simulink model "Simulink_Control_BlueROV_Modo_Deslizante"  (R2019a)
settings: Solver=VariableStepAuto  StartTime=0.0  StopTime=100*3  RelTol=1e-3
values from neighbouring files (symbols this model uses):
  a0 = 50    [Control_BlueROV_Modo_Deslizante.m]
  a1 = 1    [Control_BlueROV_Modo_Deslizante.m]
  B = 78.38    [Control_BlueROV_Modo_Deslizante.m]
  eta = 1    [Control_BlueROV_Modo_Deslizante.m]
  Ix = 0.16    [Control_BlueROV_Modo_Deslizante.m]
  Ixy = 0    [Control_BlueROV_Modo_Deslizante.m]
  Ixz = 0    [Control_BlueROV_Modo_Deslizante.m]
  Iy = 0.16    [Control_BlueROV_Modo_Deslizante.m]
  Iyz = 0    [Control_BlueROV_Modo_Deslizante.m]
  Iz = 0.16    [Control_BlueROV_Modo_Deslizante.m]
  Kp = -0.07    [Control_BlueROV_Modo_Deslizante.m]
  Kpdot = -0.12    [Control_BlueROV_Modo_Deslizante.m]
  Kpp = -1.55    [Control_BlueROV_Modo_Deslizante.m]
  m = 7.31    [Control_BlueROV_Modo_Deslizante.m]
  M = Mrb+Ma    [Control_BlueROV_Modo_Deslizante.m]
  Minv = inv(M)    [Control_BlueROV_Modo_Deslizante.m]
  Mq = -0.07    [Control_BlueROV_Modo_Deslizante.m]
  Mqdot = -0.12    [Control_BlueROV_Modo_Deslizante.m]
  Mqq = -1.55    [Control_BlueROV_Modo_Deslizante.m]
  Nr = -0.07    [Control_BlueROV_Modo_Deslizante.m]
  Nrdot = -0.12    [Control_BlueROV_Modo_Deslizante.m]
  Nrr = -1.55    [Control_BlueROV_Modo_Deslizante.m]
  W = 71.71    [Control_BlueROV_Modo_Deslizante.m]
  xb = 0    [Control_BlueROV_Modo_Deslizante.m]
  xg = 0    [Control_BlueROV_Modo_Deslizante.m]
  Xu = -4.03    [Control_BlueROV_Modo_Deslizante.m]
  Xudot = -5.5    [Control_BlueROV_Modo_Deslizante.m]
  Xuu = -18.18    [Control_BlueROV_Modo_Deslizante.m]
  yb = 0    [Control_BlueROV_Modo_Deslizante.m]
  yg = 0    [Control_BlueROV_Modo_Deslizante.m]
  Yv = -6.22    [Control_BlueROV_Modo_Deslizante.m]
  Yvdot = -12.7    [Control_BlueROV_Modo_Deslizante.m]
  Yvv = -21.66    [Control_BlueROV_Modo_Deslizante.m]
  zb = 0.00019    [Control_BlueROV_Modo_Deslizante.m]
  zg = 0    [Control_BlueROV_Modo_Deslizante.m]
  Zw = -5.18    [Control_BlueROV_Modo_Deslizante.m]
  Zwdot = -14.57    [Control_BlueROV_Modo_Deslizante.m]
  Zww = -36.99    [Control_BlueROV_Modo_Deslizante.m]
(part 2 of 2)

== system Simulink_Control_BlueROV_Modo_Deslizante/BlueRov2/C(v)/Subsystem22 ==
  In1 : Inport
  In2 : Inport  Port=2
  In3 : Inport  Port=3
  In4 : Inport  Port=4
  Add4 : Sum  Inputs=+++
  Add8 : Sum
  Constant : Constant  Value=-Iyz
  Constant1 : Constant  Value=Iy
  Constant10 : Constant  Value=-Ixy
  Constant11 : Constant  Value=-Mqdot
  Product{1,19..21} (4 alike) : Product
  Out1 : Outport
  wires:
  In2/1 -> Product20/2
  In1/1 -> Product19/2
  Add8/1 -> Out1/1
  Constant10/1 -> Product20/1
  Product21/1 -> Add8/2
  Constant/1 -> Product19/1
  Product19/1 -> Add4/1
  Add4/1 -> Add8/1
  Constant11/1 -> Product21/1
  Product20/1 -> Add4/2
  Product1/1 -> Add4/3
  Constant1/1 -> Product1/1
  In4/1 -> Product21/2
  In3/1 -> Product1/2

== system Simulink_Control_BlueROV_Modo_Deslizante/BlueRov2/C(v)/Subsystem23 ==
  In1 : Inport
  In2 : Inport  Port=2
  In3 : Inport  Port=3
  In4 : Inport  Port=4
  Add4 : Sum  Inputs=+++
  Add8 : Sum
  Constant : Constant  Value=Ixz
  Constant1 : Constant  Value=-Ix
  Constant10 : Constant  Value=Ixy
  Constant11 : Constant  Value=Kpdot
  Product{1,19..21} (4 alike) : Product
  Out1 : Outport
  wires:
  In3/1 -> Product1/2
  In4/1 -> Product21/2
  Constant1/1 -> Product1/1
  Product1/1 -> Add4/3
  Product20/1 -> Add4/2
  Constant11/1 -> Product21/1
  Add4/1 -> Add8/1
  Product19/1 -> Add4/1
  Constant/1 -> Product19/1
  Product21/1 -> Add8/2
  Constant10/1 -> Product20/1
  Add8/1 -> Out1/1
  In1/1 -> Product19/2
  In2/1 -> Product20/2

== system Simulink_Control_BlueROV_Modo_Deslizante/BlueRov2/C(v)/Subsystem3 ==
  In1 : Inport
  In2 : Inport  Port=2
  In3 : Inport  Port=3
  Add4 : Sum
  Add8 : Sum  Inputs=-+
  Constant : Constant  Value=yg
  Constant10 : Constant
  Constant11 : Constant  Value=Zwdot
  Gain : Gain  Gain=m
  Product19 : Product
  Product20 : Product
  Product21 : Product
  Out1 : Outport
  wires:
  In2/1 -> Product20/2
  In3/1 -> Product21/2
  In1/1 -> Product19/2
  Add8/1 -> Out1/1
  Constant10/1 -> Product20/1
  Add4/1 -> Gain/1
  Product21/1 -> Add8/2
  Constant/1 -> Product19/1
  Product19/1 -> Add4/1
  Gain/1 -> Add8/1
  Constant11/1 -> Product21/1
  Product20/1 -> Add4/2

== system Simulink_Control_BlueROV_Modo_Deslizante/BlueRov2/C(v)/Subsystem4 ==
  In1 : Inport
  In2 : Inport  Port=2
  Add4 : Sum
  Constant : Constant  Value=zg
  Constant10 : Constant  Value=xg
  Gain : Gain  Gain=m
  Product19 : Product
  Product20 : Product
  Out1 : Outport
  wires:
  In2/1 -> Product20/2
  Add4/1 -> Gain/1
  Constant10/1 -> Product20/1
  Gain/1 -> Out1/1
  Constant/1 -> Product19/1
  In1/1 -> Product19/2
  Product19/1 -> Add4/1
  Product20/1 -> Add4/2

== system Simulink_Control_BlueROV_Modo_Deslizante/BlueRov2/C(v)/Subsystem5 ==
  In1 : Inport
  In2 : Inport  Port=2
  In3 : Inport  Port=3
  Add4 : Sum  Inputs=+-
  Add8 : Sum  Inputs=-+
  Constant : Constant  Value=yg
  Constant10 : Constant
  Constant11 : Constant  Value=-Xudot
  Gain : Gain  Gain=m
  Product19 : Product
  Product20 : Product
  Product21 : Product
  Out1 : Outport
  wires:
  Product20/1 -> Add4/2
  Constant11/1 -> Product21/1
  Gain/1 -> Add8/1
  Product19/1 -> Add4/1
  Constant/1 -> Product19/1
  Product21/1 -> Add8/2
  Add4/1 -> Gain/1
  Constant10/1 -> Product20/1
  Add8/1 -> Out1/1
  In1/1 -> Product19/2
  In3/1 -> Product21/2
  In2/1 -> Product20/2

== system Simulink_Control_BlueROV_Modo_Deslizante/BlueRov2/C(v)/Subsystem6 ==
  In1 : Inport
  In2 : Inport  Port=2
  In3 : Inport  Port=3
  Add4 : Sum  Inputs=+-
  Add8 : Sum  Inputs=-+
  Constant : Constant  Value=zg
  Constant10 : Constant
  Constant11 : Constant  Value=-Yvdot
  Gain : Gain  Gain=m
  Product19 : Product
  Product20 : Product
  Product21 : Product
  Out1 : Outport
  wires:
  In2/1 -> Product20/2
  In3/1 -> Product21/2
  In1/1 -> Product19/2
  Add8/1 -> Out1/1
  Constant10/1 -> Product20/1
  Add4/1 -> Gain/1
  Product21/1 -> Add8/2
  Constant/1 -> Product19/1
  Product19/1 -> Add4/1
  Gain/1 -> Add8/1
  Constant11/1 -> Product21/1
  Product20/1 -> Add4/2

== system Simulink_Control_BlueROV_Modo_Deslizante/BlueRov2/C(v)/Subsystem7 ==
  In1 : Inport
  In2 : Inport  Port=2
  In3 : Inport  Port=3
  Add4 : Sum
  Add8 : Sum  Inputs=-+
  Constant : Constant  Value=zg
  Constant10 : Constant
  Constant11 : Constant  Value=Xudot
  Gain : Gain  Gain=m
  Product19 : Product
  Product20 : Product
  Product21 : Product
  Out1 : Outport
  wires:
  Product20/1 -> Add4/2
  Constant11/1 -> Product21/1
  Gain/1 -> Add8/1
  Product19/1 -> Add4/1
  Constant/1 -> Product19/1
  Product21/1 -> Add8/2
  Add4/1 -> Gain/1
  Constant10/1 -> Product20/1
  Add8/1 -> Out1/1
  In1/1 -> Product19/2
  In3/1 -> Product21/2
  In2/1 -> Product20/2

== system Simulink_Control_BlueROV_Modo_Deslizante/BlueRov2/C(v)/Subsystem8 ==
  In1 : Inport
  In2 : Inport  Port=2
  Add4 : Sum
  Constant : Constant  Value=xg
  Constant10 : Constant  Value=yg
  Gain : Gain  Gain=m
  Product19 : Product
  Product20 : Product
  Out1 : Outport
  wires:
  In2/1 -> Product20/2
  Add4/1 -> Gain/1
  Constant10/1 -> Product20/1
  Gain/1 -> Out1/1
  Constant/1 -> Product19/1
  In1/1 -> Product19/2
  Product19/1 -> Add4/1
  Product20/1 -> Add4/2

== system Simulink_Control_BlueROV_Modo_Deslizante/BlueRov2/C(v)/Subsystem9 ==
  In1 : Inport
  In2 : Inport  Port=2
  Add4 : Sum
  Constant : Constant  Value=yg
  Constant10 : Constant  Value=zg
  Gain : Gain  Gain=-m
  Product19 : Product
  Product20 : Product
  Out1 : Outport
  wires:
  In2/1 -> Product20/2
  Add4/1 -> Gain/1
  Constant10/1 -> Product20/1
  Gain/1 -> Out1/1
  Constant/1 -> Product19/1
  In1/1 -> Product19/2
  Product19/1 -> Add4/1
  Product20/1 -> Add4/2

== system Simulink_Control_BlueROV_Modo_Deslizante/BlueRov2/J(n)/Subsystem1 ==
  In1 : Inport
  In2 : Inport  Port=2
  Product6 : Product
  Out1 : Outport
  wires:
  In1/1 -> Product6/1
  In2/1 -> Product6/2
  Product6/1 -> Out1/1

== system Simulink_Control_BlueROV_Modo_Deslizante/BlueRov2/J(n)/Subsystem10 ==
  In1 : Inport
  In2 : Inport  Port=2
  Product6 : Product
  Out1 : Outport
  wires:
  In1/1 -> Product6/1
  In2/1 -> Product6/2
  Product6/1 -> Out1/1

== system Simulink_Control_BlueROV_Modo_Deslizante/BlueRov2/J(n)/Subsystem11 ==
  In1 : Inport
  In2 : Inport  Port=2
  Product6 : Product
  Out1 : Outport
  wires:
  In1/1 -> Product6/1
  In2/1 -> Product6/2
  Product6/1 -> Out1/1

== system Simulink_Control_BlueROV_Modo_Deslizante/BlueRov2/J(n)/Subsystem12 ==
  In1 : Inport
  In2 : Inport  Port=2
  Product6 : Product
  Out1 : Outport
  wires:
  In1/1 -> Product6/1
  In2/1 -> Product6/2
  Product6/1 -> Out1/1

== system Simulink_Control_BlueROV_Modo_Deslizante/BlueRov2/J(n)/Subsystem2 ==
  In1 : Inport
  In2 : Inport  Port=2
  In3 : Inport  Port=3
  In4 : Inport  Port=4
  In5 : Inport  Port=5
  Add7 : Sum
  Product37 : Product
  Product38 : Product  Inputs=3
  Out1 : Outport
  wires:
  In5/1 -> Product38/3
  In4/1 -> Product38/2
  In3/1 -> Product38/1
  In2/1 -> Product37/2
  In1/1 -> Product37/1
  Product37/1 -> Add7/1
  Add7/1 -> Out1/1
  Product38/1 -> Add7/2

== system Simulink_Control_BlueROV_Modo_Deslizante/BlueRov2/J(n)/Subsystem3 ==
  In1 : Inport
  In2 : Inport  Port=2
  Product6 : Product
  Out1 : Outport
  wires:
  Product6/1 -> Out1/1
  In2/1 -> Product6/2
  In1/1 -> Product6/1

== system Simulink_Control_BlueROV_Modo_Deslizante/BlueRov2/J(n)/Subsystem4 ==
  In1 : Inport
  In2 : Inport  Port=2
  In3 : Inport  Port=3
  In4 : Inport  Port=4
  In5 : Inport  Port=5
  Add7 : Sum  Inputs=-+
  Product37 : Product
  Product38 : Product  Inputs=3
  Out1 : Outport
  wires:
  Product38/1 -> Add7/2
  Add7/1 -> Out1/1
  Product37/1 -> Add7/1
  In1/1 -> Product37/1
  In2/1 -> Product37/2
  In3/1 -> Product38/1
  In4/1 -> Product38/2
  In5/1 -> Product38/3

== system Simulink_Control_BlueROV_Modo_Deslizante/BlueRov2/J(n)/Subsystem5 ==
  In1 : Inport
  In2 : Inport  Port=2
  In3 : Inport  Port=3
  In4 : Inport  Port=4
  In5 : Inport  Port=5
  Add7 : Sum
  Product37 : Product
  Product38 : Product  Inputs=3
  Out1 : Outport
  wires:
  Product38/1 -> Add7/2
  Add7/1 -> Out1/1
  Product37/1 -> Add7/1
  In1/1 -> Product37/1
  In2/1 -> Product37/2
  In3/1 -> Product38/1
  In4/1 -> Product38/2
  In5/1 -> Product38/3

== system Simulink_Control_BlueROV_Modo_Deslizante/BlueRov2/J(n)/Subsystem6 ==
  In1 : Inport
  In2 : Inport  Port=2
  In3 : Inport  Port=3
  In4 : Inport  Port=4
  In5 : Inport  Port=5
  Add7 : Sum  Inputs=-+
  Product37 : Product
  Product38 : Product  Inputs=3
  Out1 : Outport
  wires:
  In5/1 -> Product38/3
  In4/1 -> Product38/2
  In3/1 -> Product38/1
  In2/1 -> Product37/2
  In1/1 -> Product37/1
  Product37/1 -> Add7/1
  Add7/1 -> Out1/1
  Product38/1 -> Add7/2

== system Simulink_Control_BlueROV_Modo_Deslizante/BlueRov2/J(n)/Subsystem7 ==
  In1 : Inport
  In2 : Inport  Port=2
  Product6 : Product
  Out1 : Outport
  wires:
  In1/1 -> Product6/1
  In2/1 -> Product6/2
  Product6/1 -> Out1/1

== system Simulink_Control_BlueROV_Modo_Deslizante/BlueRov2/J(n)/Subsystem8 ==
  In1 : Inport
  In2 : Inport  Port=2
  Product6 : Product
  Out1 : Outport
  wires:
  Product6/1 -> Out1/1
  In2/1 -> Product6/2
  In1/1 -> Product6/1

== system Simulink_Control_BlueROV_Modo_Deslizante/BlueRov2/J(n)/Subsystem9 ==
  In1 : Inport
  In2 : Inport  Port=2
  Product6 : Product
  Out1 : Outport
  wires:
  In1/1 -> Product6/1
  In2/1 -> Product6/2
  Product6/1 -> Out1/1

== system Simulink_Control_BlueROV_Modo_Deslizante/Estimador de Variable/C(v)/Subsystem ==
  In1 : Inport
  In2 : Inport  Port=2
  Add4 : Sum
  Constant : Constant  Value=zg
  Constant10 : Constant  Value=yg
  Gain : Gain  Gain=m
  Product19 : Product
  Product20 : Product
  Out1 : Outport
  wires:
  Product20/1 -> Add4/2
  Product19/1 -> Add4/1
  In1/1 -> Product19/2
  Constant/1 -> Product19/1
  Gain/1 -> Out1/1
  Constant10/1 -> Product20/1
  Add4/1 -> Gain/1
  In2/1 -> Product20/2

== system Simulink_Control_BlueROV_Modo_Deslizante/Estimador de Variable/C(v)/Subsystem1 ==
  In1 : Inport
  In2 : Inport  Port=2
  In3 : Inport  Port=3
  Add4 : Sum  Inputs=+-
  Add8 : Sum  Inputs=-+
  Constant : Constant  Value=xg
  Constant10 : Constant
  Constant11 : Constant  Value=-Zwdot
  Gain : Gain  Gain=m
  Product19 : Product
  Product20 : Product
  Product21 : Product
  Out1 : Outport
  wires:
  Product20/1 -> Add4/2
  Constant11/1 -> Product21/1
  Gain/1 -> Add8/1
  Product19/1 -> Add4/1
  Constant/1 -> Product19/1
  Product21/1 -> Add8/2
  Add4/1 -> Gain/1
  Constant10/1 -> Product20/1
  Add8/1 -> Out1/1
  In1/1 -> Product19/2
  In3/1 -> Product21/2
  In2/1 -> Product20/2

== system Simulink_Control_BlueROV_Modo_Deslizante/Estimador de Variable/C(v)/Subsystem10 ==
  In1 : Inport
  In2 : Inport  Port=2
  In3 : Inport  Port=3
  Add4 : Sum
  Add8 : Sum
  Constant : Constant  Value=yg
  Constant10 : Constant
  Constant11 : Constant  Value=-Zwdot
  Gain : Gain  Gain=m
  Product19 : Product
  Product20 : Product
  Product21 : Product
  Out1 : Outport
  wires:
  In2/1 -> Product20/2
  In3/1 -> Product21/2
  In1/1 -> Product19/2
  Add8/1 -> Out1/1
  Constant10/1 -> Product20/1
  Add4/1 -> Gain/1
  Product21/1 -> Add8/2
  Constant/1 -> Product19/1
  Product19/1 -> Add4/1
  Gain/1 -> Add8/1
  Constant11/1 -> Product21/1
  Product20/1 -> Add4/2

== system Simulink_Control_BlueROV_Modo_Deslizante/Estimador de Variable/C(v)/Subsystem11 ==
  In1 : Inport
  In2 : Inport  Port=2
  In3 : Inport  Port=3
  Add4 : Sum  Inputs=+-
  Add8 : Sum
  Constant : Constant  Value=zg
  Constant10 : Constant
  Constant11 : Constant  Value=Yvdot
  Gain : Gain  Gain=m
  Product19 : Product
  Product20 : Product
  Product21 : Product
  Out1 : Outport
  wires:
  Product20/1 -> Add4/2
  Constant11/1 -> Product21/1
  Gain/1 -> Add8/1
  Product19/1 -> Add4/1
  Constant/1 -> Product19/1
  Product21/1 -> Add8/2
  Add4/1 -> Gain/1
  Constant10/1 -> Product20/1
  Add8/1 -> Out1/1
  In1/1 -> Product19/2
  In3/1 -> Product21/2
  In2/1 -> Product20/2

== system Simulink_Control_BlueROV_Modo_Deslizante/Estimador de Variable/C(v)/Subsystem12 ==
  In1 : Inport
  In2 : Inport  Port=2
  In3 : Inport  Port=3
  In4 : Inport  Port=4
  Add4 : Sum  Inputs=+++
  Add8 : Sum
  Constant : Constant  Value=-Iyz
  Constant1 : Constant  Value=Iz
  Constant10 : Constant  Value=-Ixz
  Constant11 : Constant  Value=-Nrdot
  Product{1,19..21} (4 alike) : Product
  Out1 : Outport
  wires:
  In2/1 -> Product20/2
  In1/1 -> Product19/2
  Add8/1 -> Out1/1
  Constant10/1 -> Product20/1
  Product21/1 -> Add8/2
  Constant/1 -> Product19/1
  Product19/1 -> Add4/1
  Add4/1 -> Add8/1
  Constant11/1 -> Product21/1
  Product20/1 -> Add4/2
  Product1/1 -> Add4/3
  Constant1/1 -> Product1/1
  In4/1 -> Product21/2
  In3/1 -> Product1/2

== system Simulink_Control_BlueROV_Modo_Deslizante/Estimador de Variable/C(v)/Subsystem13 ==
  In1 : Inport
  In2 : Inport  Port=2
  In3 : Inport  Port=3
  In4 : Inport  Port=4
  Add4 : Sum  Inputs=+++
  Add8 : Sum
  Constant : Constant  Value=Iyz
  Constant1 : Constant  Value=-Iy
  Constant10 : Constant  Value=Ixy
  Constant11 : Constant  Value=Mqdot
  Product{1,19..21} (4 alike) : Product
  Out1 : Outport
  wires:
  In3/1 -> Product1/2
  In4/1 -> Product21/2
  Constant1/1 -> Product1/1
  Product1/1 -> Add4/3
  Product20/1 -> Add4/2
  Constant11/1 -> Product21/1
  Add4/1 -> Add8/1
  Product19/1 -> Add4/1
  Constant/1 -> Product19/1
  Product21/1 -> Add8/2
  Constant10/1 -> Product20/1
  Add8/1 -> Out1/1
  In1/1 -> Product19/2
  In2/1 -> Product20/2

== system Simulink_Control_BlueROV_Modo_Deslizante/Estimador de Variable/C(v)/Subsystem14 ==
  In1 : Inport
  In2 : Inport  Port=2
  In3 : Inport  Port=3
  Add4 : Sum  Inputs=+-
  Add8 : Sum
  Constant : Constant  Value=xg
  Constant10 : Constant
  Constant11 : Constant  Value=Zwdot
  Gain : Gain  Gain=m
  Product19 : Product
  Product20 : Product
  Product21 : Product
  Out1 : Outport
  wires:
  Product20/1 -> Add4/2
  Constant11/1 -> Product21/1
  Gain/1 -> Add8/1
  Product19/1 -> Add4/1
  Constant/1 -> Product19/1
  Product21/1 -> Add8/2
  Add4/1 -> Gain/1
  Constant10/1 -> Product20/1
  Add8/1 -> Out1/1
  In1/1 -> Product19/2
  In3/1 -> Product21/2
  In2/1 -> Product20/2

== system Simulink_Control_BlueROV_Modo_Deslizante/Estimador de Variable/C(v)/Subsystem15 ==
  In1 : Inport
  In2 : Inport  Port=2
  In3 : Inport  Port=3
  Add4 : Sum
  Add8 : Sum
  Constant : Constant  Value=zg
  Constant10 : Constant
  Constant11 : Constant  Value=-Xudot
  Gain : Gain  Gain=m
  Product19 : Product
  Product20 : Product
  Product21 : Product
  Out1 : Outport
  wires:
  In2/1 -> Product20/2
  In3/1 -> Product21/2
  In1/1 -> Product19/2
  Add8/1 -> Out1/1
  Constant10/1 -> Product20/1
  Add4/1 -> Gain/1
  Product21/1 -> Add8/2
  Constant/1 -> Product19/1
  Product19/1 -> Add4/1
  Gain/1 -> Add8/1
  Constant11/1 -> Product21/1
  Product20/1 -> Add4/2

== system Simulink_Control_BlueROV_Modo_Deslizante/Estimador de Variable/C(v)/Subsystem16 ==
  In1 : Inport
  In2 : Inport  Port=2
  Add4 : Sum
  Constant : Constant  Value=zg
  Constant10 : Constant  Value=xg
  Gain : Gain  Gain=-m
  Product19 : Product
  Product20 : Product
  Out1 : Outport
  wires:
  Product20/1 -> Add4/2
  Product19/1 -> Add4/1
  In1/1 -> Product19/2
  Constant/1 -> Product19/1
  Gain/1 -> Out1/1
  Constant10/1 -> Product20/1
  Add4/1 -> Gain/1
  In2/1 -> Product20/2

== system Simulink_Control_BlueROV_Modo_Deslizante/Estimador de Variable/C(v)/Subsystem17 ==
  In1 : Inport
  In2 : Inport  Port=2
  In3 : Inport  Port=3
  In4 : Inport  Port=4
  Add4 : Sum  Inputs=+++
  Add8 : Sum
  Constant : Constant  Value=Iyz
  Constant1 : Constant  Value=-Iz
  Constant10 : Constant  Value=Ixz
  Constant11 : Constant  Value=Nrdot
  Product{1,19..21} (4 alike) : Product
  Out1 : Outport
  wires:
  In3/1 -> Product1/2
  In4/1 -> Product21/2
  Constant1/1 -> Product1/1
  Product1/1 -> Add4/3
  Product20/1 -> Add4/2
  Constant11/1 -> Product21/1
  Add4/1 -> Add8/1
  Product19/1 -> Add4/1
  Constant/1 -> Product19/1
  Product21/1 -> Add8/2
  Constant10/1 -> Product20/1
  Add8/1 -> Out1/1
  In1/1 -> Product19/2
  In2/1 -> Product20/2

== system Simulink_Control_BlueROV_Modo_Deslizante/Estimador de Variable/C(v)/Subsystem18 ==
  In1 : Inport
  In2 : Inport  Port=2
  In3 : Inport  Port=3
  In4 : Inport  Port=4
  Add4 : Sum  Inputs=+++
  Add8 : Sum
  Constant : Constant  Value=-Ixz
  Constant1 : Constant  Value=Ix
  Constant10 : Constant  Value=-Ixy
  Constant11 : Constant  Value=-Kpdot
  Product{1,19..21} (4 alike) : Product
  Out1 : Outport
  wires:
  In2/1 -> Product20/2
  In1/1 -> Product19/2
  Add8/1 -> Out1/1
  Constant10/1 -> Product20/1
  Product21/1 -> Add8/2
  Constant/1 -> Product19/1
  Product19/1 -> Add4/1
  Add4/1 -> Add8/1
  Constant11/1 -> Product21/1
  Product20/1 -> Add4/2
  Product1/1 -> Add4/3
  Constant1/1 -> Product1/1
  In4/1 -> Product21/2
  In3/1 -> Product1/2

== system Simulink_Control_BlueROV_Modo_Deslizante/Estimador de Variable/C(v)/Subsystem19 ==
  In1 : Inport
  In2 : Inport  Port=2
  In3 : Inport  Port=3
  Add4 : Sum
  Add8 : Sum
  Constant : Constant  Value=xg
  Constant10 : Constant
  Constant11 : Constant  Value=-Yvdot
  Gain : Gain  Gain=m
  Product19 : Product
  Product20 : Product
  Product21 : Product
  Out1 : Outport
  wires:
  In2/1 -> Product20/2
  In3/1 -> Product21/2
  In1/1 -> Product19/2
  Add8/1 -> Out1/1
  Constant10/1 -> Product20/1
  Add4/1 -> Gain/1
  Product21/1 -> Add8/2
  Constant/1 -> Product19/1
  Product19/1 -> Add4/1
  Gain/1 -> Add8/1
  Constant11/1 -> Product21/1
  Product20/1 -> Add4/2

== system Simulink_Control_BlueROV_Modo_Deslizante/Estimador de Variable/C(v)/Subsystem2 ==
  In1 : Inport
  In2 : Inport  Port=2
  In3 : Inport  Port=3
  Add10 : Sum  Inputs=-+
  Add9 : Sum
  Constant12 : Constant  Value=xg
  Constant13 : Constant
  Constant14 : Constant  Value=Yvdot
  Gain1 : Gain  Gain=m
  Product22 : Product
  Product23 : Product
  Product24 : Product
  Out1 : Outport
  wires:
  In1/1 -> Product22/2
  Constant14/1 -> Product24/1
  Add9/1 -> Gain1/1
  Constant12/1 -> Product22/1
  Product23/1 -> Add9/2
  Gain1/1 -> Add10/1
  Constant13/1 -> Product23/1
  Product24/1 -> Add10/2
  Product22/1 -> Add9/1
  In3/1 -> Product24/2
  Add10/1 -> Out1/1
  In2/1 -> Product23/2

== system Simulink_Control_BlueROV_Modo_Deslizante/Estimador de Variable/C(v)/Subsystem20 ==
  In1 : Inport
  In2 : Inport  Port=2
  In3 : Inport  Port=3
  Add4 : Sum
  Add8 : Sum
  Constant : Constant  Value=yg
  Constant10 : Constant  Value=-1
  Constant11 : Constant  Value=Xudot
  Gain : Gain  Gain=m
  Product19 : Product
  Product20 : Product
  Product21 : Product
  Out1 : Outport
  wires:
  Product20/1 -> Add4/2
  Constant11/1 -> Product21/1
  Gain/1 -> Add8/1
  Product19/1 -> Add4/1
  Constant/1 -> Product19/1
  Product21/1 -> Add8/2
  Add4/1 -> Gain/1
  Constant10/1 -> Product20/1
  Add8/1 -> Out1/1
  In1/1 -> Product19/2
  In3/1 -> Product21/2
  In2/1 -> Product20/2

== system Simulink_Control_BlueROV_Modo_Deslizante/Estimador de Variable/C(v)/Subsystem21 ==
  In1 : Inport
  In2 : Inport  Port=2
  Add4 : Sum
  Constant : Constant  Value=xg
  Constant10 : Constant  Value=yg
  Gain : Gain  Gain=-m
  Product19 : Product
  Product20 : Product
  Out1 : Outport
  wires:
  In2/1 -> Product20/2
  Add4/1 -> Gain/1
  Constant10/1 -> Product20/1
  Gain/1 -> Out1/1
  Constant/1 -> Product19/1
  In1/1 -> Product19/2
  Product19/1 -> Add4/1
  Product20/1 -> Add4/2

== system Simulink_Control_BlueROV_Modo_Deslizante/Estimador de Variable/C(v)/Subsystem22 ==
  In1 : Inport
  In2 : Inport  Port=2
  In3 : Inport  Port=3
  In4 : Inport  Port=4
  Add4 : Sum  Inputs=+++
  Add8 : Sum
  Constant : Constant  Value=-Iyz
  Constant1 : Constant  Value=Iy
  Constant10 : Constant  Value=-Ixy
  Constant11 : Constant  Value=-Mqdot
  Product{1,19..21} (4 alike) : Product
  Out1 : Outport
  wires:
  In2/1 -> Product20/2
  In1/1 -> Product19/2
  Add8/1 -> Out1/1
  Constant10/1 -> Product20/1
  Product21/1 -> Add8/2
  Constant/1 -> Product19/1
  Product19/1 -> Add4/1
  Add4/1 -> Add8/1
  Constant11/1 -> Product21/1
  Product20/1 -> Add4/2
  Product1/1 -> Add4/3
  Constant1/1 -> Product1/1
  In4/1 -> Product21/2
  In3/1 -> Product1/2

== system Simulink_Control_BlueROV_Modo_Deslizante/Estimador de Variable/C(v)/Subsystem23 ==
  In1 : Inport
  In2 : Inport  Port=2
  In3 : Inport  Port=3
  In4 : Inport  Port=4
  Add4 : Sum  Inputs=+++
  Add8 : Sum
  Constant : Constant  Value=Ixz
  Constant1 : Constant  Value=-Ix
  Constant10 : Constant  Value=Ixy
  Constant11 : Constant  Value=Kpdot
  Product{1,19..21} (4 alike) : Product
  Out1 : Outport
  wires:
  In3/1 -> Product1/2
  In4/1 -> Product21/2
  Constant1/1 -> Product1/1
  Product1/1 -> Add4/3
  Product20/1 -> Add4/2
  Constant11/1 -> Product21/1
  Add4/1 -> Add8/1
  Product19/1 -> Add4/1
  Constant/1 -> Product19/1
  Product21/1 -> Add8/2
  Constant10/1 -> Product20/1
  Add8/1 -> Out1/1
  In1/1 -> Product19/2
  In2/1 -> Product20/2

== system Simulink_Control_BlueROV_Modo_Deslizante/Estimador de Variable/C(v)/Subsystem3 ==
  In1 : Inport
  In2 : Inport  Port=2
  In3 : Inport  Port=3
  Add4 : Sum
  Add8 : Sum  Inputs=-+
  Constant : Constant  Value=yg
  Constant10 : Constant
  Constant11 : Constant  Value=Zwdot
  Gain : Gain  Gain=m
  Product19 : Product
  Product20 : Product
  Product21 : Product
  Out1 : Outport
  wires:
  In2/1 -> Product20/2
  In3/1 -> Product21/2
  In1/1 -> Product19/2
  Add8/1 -> Out1/1
  Constant10/1 -> Product20/1
  Add4/1 -> Gain/1
  Product21/1 -> Add8/2
  Constant/1 -> Product19/1
  Product19/1 -> Add4/1
  Gain/1 -> Add8/1
  Constant11/1 -> Product21/1
  Product20/1 -> Add4/2

== system Simulink_Control_BlueROV_Modo_Deslizante/Estimador de Variable/C(v)/Subsystem4 ==
  In1 : Inport
  In2 : Inport  Port=2
  Add4 : Sum
  Constant : Constant  Value=zg
  Constant10 : Constant  Value=xg
  Gain : Gain  Gain=m
  Product19 : Product
  Product20 : Product
  Out1 : Outport
  wires:
  In2/1 -> Product20/2
  Add4/1 -> Gain/1
  Constant10/1 -> Product20/1
  Gain/1 -> Out1/1
  Constant/1 -> Product19/1
  In1/1 -> Product19/2
  Product19/1 -> Add4/1
  Product20/1 -> Add4/2

== system Simulink_Control_BlueROV_Modo_Deslizante/Estimador de Variable/C(v)/Subsystem5 ==
  In1 : Inport
  In2 : Inport  Port=2
  In3 : Inport  Port=3
  Add4 : Sum  Inputs=+-
  Add8 : Sum  Inputs=-+
  Constant : Constant  Value=yg
  Constant10 : Constant
  Constant11 : Constant  Value=-Xudot
  Gain : Gain  Gain=m
  Product19 : Product
  Product20 : Product
  Product21 : Product
  Out1 : Outport
  wires:
  Product20/1 -> Add4/2
  Constant11/1 -> Product21/1
  Gain/1 -> Add8/1
  Product19/1 -> Add4/1
  Constant/1 -> Product19/1
  Product21/1 -> Add8/2
  Add4/1 -> Gain/1
  Constant10/1 -> Product20/1
  Add8/1 -> Out1/1
  In1/1 -> Product19/2
  In3/1 -> Product21/2
  In2/1 -> Product20/2

== system Simulink_Control_BlueROV_Modo_Deslizante/Estimador de Variable/C(v)/Subsystem6 ==
  In1 : Inport
  In2 : Inport  Port=2
  In3 : Inport  Port=3
  Add4 : Sum  Inputs=+-
  Add8 : Sum  Inputs=-+
  Constant : Constant  Value=zg
  Constant10 : Constant
  Constant11 : Constant  Value=-Yvdot
  Gain : Gain  Gain=m
  Product19 : Product
  Product20 : Product
  Product21 : Product
  Out1 : Outport
  wires:
  In2/1 -> Product20/2
  In3/1 -> Product21/2
  In1/1 -> Product19/2
  Add8/1 -> Out1/1
  Constant10/1 -> Product20/1
  Add4/1 -> Gain/1
  Product21/1 -> Add8/2
  Constant/1 -> Product19/1
  Product19/1 -> Add4/1
  Gain/1 -> Add8/1
  Constant11/1 -> Product21/1
  Product20/1 -> Add4/2

== system Simulink_Control_BlueROV_Modo_Deslizante/Estimador de Variable/C(v)/Subsystem7 ==
  In1 : Inport
  In2 : Inport  Port=2
  In3 : Inport  Port=3
  Add4 : Sum
  Add8 : Sum  Inputs=-+
  Constant : Constant  Value=zg
  Constant10 : Constant
  Constant11 : Constant  Value=Xudot
  Gain : Gain  Gain=m
  Product19 : Product
  Product20 : Product
  Product21 : Product
  Out1 : Outport
  wires:
  Product20/1 -> Add4/2
  Constant11/1 -> Product21/1
  Gain/1 -> Add8/1
  Product19/1 -> Add4/1
  Constant/1 -> Product19/1
  Product21/1 -> Add8/2
  Add4/1 -> Gain/1
  Constant10/1 -> Product20/1
  Add8/1 -> Out1/1
  In1/1 -> Product19/2
  In3/1 -> Product21/2
  In2/1 -> Product20/2

== system Simulink_Control_BlueROV_Modo_Deslizante/Estimador de Variable/C(v)/Subsystem8 ==
  In1 : Inport
  In2 : Inport  Port=2
  Add4 : Sum
  Constant : Constant  Value=xg
  Constant10 : Constant  Value=yg
  Gain : Gain  Gain=m
  Product19 : Product
  Product20 : Product
  Out1 : Outport
  wires:
  In2/1 -> Product20/2
  Add4/1 -> Gain/1
  Constant10/1 -> Product20/1
  Gain/1 -> Out1/1
  Constant/1 -> Product19/1
  In1/1 -> Product19/2
  Product19/1 -> Add4/1
  Product20/1 -> Add4/2

== system Simulink_Control_BlueROV_Modo_Deslizante/Estimador de Variable/C(v)/Subsystem9 ==
  In1 : Inport
  In2 : Inport  Port=2
  Add4 : Sum
  Constant : Constant  Value=yg
  Constant10 : Constant  Value=zg
  Gain : Gain  Gain=-m
  Product19 : Product
  Product20 : Product
  Out1 : Outport
  wires:
  In2/1 -> Product20/2
  Add4/1 -> Gain/1
  Constant10/1 -> Product20/1
  Gain/1 -> Out1/1
  Constant/1 -> Product19/1
  In1/1 -> Product19/2
  Product19/1 -> Add4/1
  Product20/1 -> Add4/2

== system Simulink_Control_BlueROV_Modo_Deslizante/Estimador de Variable/J(n)/Subsystem1 ==
  In1 : Inport
  In2 : Inport  Port=2
  Product6 : Product
  Out1 : Outport
  wires:
  In1/1 -> Product6/1
  In2/1 -> Product6/2
  Product6/1 -> Out1/1

== system Simulink_Control_BlueROV_Modo_Deslizante/Estimador de Variable/J(n)/Subsystem10 ==
  In1 : Inport
  In2 : Inport  Port=2
  Product6 : Product
  Out1 : Outport
  wires:
  In1/1 -> Product6/1
  In2/1 -> Product6/2
  Product6/1 -> Out1/1

== system Simulink_Control_BlueROV_Modo_Deslizante/Estimador de Variable/J(n)/Subsystem11 ==
  In1 : Inport
  In2 : Inport  Port=2
  Product6 : Product
  Out1 : Outport
  wires:
  In1/1 -> Product6/1
  In2/1 -> Product6/2
  Product6/1 -> Out1/1

== system Simulink_Control_BlueROV_Modo_Deslizante/Estimador de Variable/J(n)/Subsystem12 ==
  In1 : Inport
  In2 : Inport  Port=2
  Product6 : Product
  Out1 : Outport
  wires:
  In1/1 -> Product6/1
  In2/1 -> Product6/2
  Product6/1 -> Out1/1

== system Simulink_Control_BlueROV_Modo_Deslizante/Estimador de Variable/J(n)/Subsystem2 ==
  In1 : Inport
  In2 : Inport  Port=2
  In3 : Inport  Port=3
  In4 : Inport  Port=4
  In5 : Inport  Port=5
  Add7 : Sum
  Product37 : Product
  Product38 : Product  Inputs=3
  Out1 : Outport
  wires:
  In5/1 -> Product38/3
  In4/1 -> Product38/2
  In3/1 -> Product38/1
  In2/1 -> Product37/2
  In1/1 -> Product37/1
  Product37/1 -> Add7/1
  Add7/1 -> Out1/1
  Product38/1 -> Add7/2

== system Simulink_Control_BlueROV_Modo_Deslizante/Estimador de Variable/J(n)/Subsystem3 ==
  In1 : Inport
  In2 : Inport  Port=2
  Product6 : Product
  Out1 : Outport
  wires:
  Product6/1 -> Out1/1
  In2/1 -> Product6/2
  In1/1 -> Product6/1

== system Simulink_Control_BlueROV_Modo_Deslizante/Estimador de Variable/J(n)/Subsystem4 ==
  In1 : Inport
  In2 : Inport  Port=2
  In3 : Inport  Port=3
  In4 : Inport  Port=4
  In5 : Inport  Port=5
  Add7 : Sum  Inputs=-+
  Product37 : Product
  Product38 : Product  Inputs=3
  Out1 : Outport
  wires:
  Product38/1 -> Add7/2
  Add7/1 -> Out1/1
  Product37/1 -> Add7/1
  In1/1 -> Product37/1
  In2/1 -> Product37/2
  In3/1 -> Product38/1
  In4/1 -> Product38/2
  In5/1 -> Product38/3

== system Simulink_Control_BlueROV_Modo_Deslizante/Estimador de Variable/J(n)/Subsystem5 ==
  In1 : Inport
  In2 : Inport  Port=2
  In3 : Inport  Port=3
  In4 : Inport  Port=4
  In5 : Inport  Port=5
  Add7 : Sum
  Product37 : Product
  Product38 : Product  Inputs=3
  Out1 : Outport
  wires:
  Product38/1 -> Add7/2
  Add7/1 -> Out1/1
  Product37/1 -> Add7/1
  In1/1 -> Product37/1
  In2/1 -> Product37/2
  In3/1 -> Product38/1
  In4/1 -> Product38/2
  In5/1 -> Product38/3

== system Simulink_Control_BlueROV_Modo_Deslizante/Estimador de Variable/J(n)/Subsystem6 ==
  In1 : Inport
  In2 : Inport  Port=2
  In3 : Inport  Port=3
  In4 : Inport  Port=4
  In5 : Inport  Port=5
  Add7 : Sum  Inputs=-+
  Product37 : Product
  Product38 : Product  Inputs=3
  Out1 : Outport
  wires:
  In5/1 -> Product38/3
  In4/1 -> Product38/2
  In3/1 -> Product38/1
  In2/1 -> Product37/2
  In1/1 -> Product37/1
  Product37/1 -> Add7/1
  Add7/1 -> Out1/1
  Product38/1 -> Add7/2

== system Simulink_Control_BlueROV_Modo_Deslizante/Estimador de Variable/J(n)/Subsystem7 ==
  In1 : Inport
  In2 : Inport  Port=2
  Product6 : Product
  Out1 : Outport
  wires:
  In1/1 -> Product6/1
  In2/1 -> Product6/2
  Product6/1 -> Out1/1

== system Simulink_Control_BlueROV_Modo_Deslizante/Estimador de Variable/J(n)/Subsystem8 ==
  In1 : Inport
  In2 : Inport  Port=2
  Product6 : Product
  Out1 : Outport
  wires:
  Product6/1 -> Out1/1
  In2/1 -> Product6/2
  In1/1 -> Product6/1

== system Simulink_Control_BlueROV_Modo_Deslizante/Estimador de Variable/J(n)/Subsystem9 ==
  In1 : Inport
  In2 : Inport  Port=2
  Product6 : Product
  Out1 : Outport
  wires:
  In1/1 -> Product6/1
  In2/1 -> Product6/2
  Product6/1 -> Out1/1

== matlab function Simulink_Control_BlueROV_Modo_Deslizante/Modo deslizante/Inv(J(n)) ==
  data: phi input; y output; theta input; psi input
function y = fcn(phi,theta,psi)

y = [((((sin(phi)*sin(psi) + sin(theta)*cos(phi)*cos(psi))*sin(theta) + cos(phi)*cos(psi)*cos(theta)^2)*((sin(phi)*sin(psi)*sin(theta) + cos(phi)*cos(psi))*cos(psi)*cos(theta) - (sin(phi)*sin(theta)*cos(psi) - sin(psi)*cos(phi))*sin(psi)*cos(theta)) - ((sin(phi)*sin(theta)*cos(psi) - sin(psi)*cos(phi))*sin(theta) + sin(phi)*cos(psi)*cos(theta)^2)*(-(sin(phi)*sin(psi) + sin(theta)*cos(phi)*cos(psi))*sin(psi)*cos(theta) + (-sin(phi)*cos(psi) + sin(psi)*sin(theta)*cos(phi))*cos(psi)*cos(theta)))*(sin(phi)*sin(psi)*sin(theta) + cos(phi)*cos(psi))*cos(psi)*cos(theta) - ((sin(phi)*sin(psi) + sin(theta)*cos(phi)*cos(psi))*((sin(phi)*sin(psi)*sin(theta) + cos(phi)*cos(psi))*cos(psi)*cos(theta) - (sin(phi)*sin(theta)*cos(psi) - sin(psi)*cos(phi))*sin(psi)*cos(theta)) - (-(sin(phi)*sin(psi) + sin(theta)*cos(phi)*cos(psi))*sin(psi)*cos(theta) + (-sin(phi)*cos(psi) + sin(psi)*sin(theta)*cos(phi))*cos(psi)*cos(theta))*(sin(phi)*sin(theta)*cos(psi) - sin(psi)*cos(phi)))*(((sin(phi)*sin(theta)*cos(psi) - sin(psi)*cos(phi))*sin(theta) + sin(phi)*cos(psi)*cos(theta)^2)*sin(psi)*cos(theta) + ((sin(phi)*sin(psi)*sin(theta) + cos(phi)*cos(psi))*cos(psi)*cos(theta) - (sin(phi)*sin(theta)*cos(psi) - sin(psi)*cos(phi))*sin(psi)*cos(theta))*sin(theta)))/((((sin(phi)*sin(psi) + sin(theta)*cos(phi)*cos(psi))*sin(theta) + cos(phi)*cos(psi)*cos(theta)^2)*((sin(phi)*sin(psi)*sin(theta) + cos(phi)*cos(psi))*cos(psi)*cos(theta) - (sin(phi)*sin(theta)*cos(psi) - sin(psi)*cos(phi))*sin(psi)*cos(theta)) - ((sin(phi)*sin(theta)*cos(psi) - sin(psi)*cos(phi))*sin(theta) + sin(phi)*cos(psi)*cos(theta)^2)*(-(sin(phi)*sin(psi) + sin(theta)*cos(phi)*cos(psi))*sin(psi)*cos(theta) + (-sin(phi)*cos(psi) + sin(psi)*sin(theta)*cos(phi))*cos(psi)*cos(theta)))*((sin(phi)*sin(psi)*sin(theta) + cos(phi)*cos(psi))*cos(psi)*cos(theta) - (sin(phi)*sin(theta)*cos(psi) - sin(psi)*cos(phi))*sin(psi)*cos(theta))*cos(psi)*cos(theta)), (-(((sin(phi)*sin(psi) + sin(theta)*cos(phi)*cos(psi))*sin(theta) + cos(phi)*cos(psi)*cos(theta)^2)*((sin(phi)*sin(psi)*sin(theta) + cos(phi)*cos(psi))*cos(psi)*cos(theta) - (sin(phi)*sin(theta)*cos(psi) - sin(psi)*cos(phi))*sin(psi)*cos(theta)) - ((sin(phi)*sin(theta)*cos(psi) - sin(psi)*cos(phi))*sin(theta) + sin(phi)*cos(psi)*cos(theta)^2)*(-(sin(phi)*sin(psi) + sin(theta)*cos(phi)*cos(psi))*sin(psi)*cos(theta) + (-sin(phi)*cos(psi) + sin(psi)*sin(theta)*cos(phi))*cos(psi)*cos(theta)))*(sin(phi)*sin(theta)*cos(psi) - sin(psi)*cos(phi))*cos(psi)*cos(theta) + ((sin(phi)*sin(psi) + sin(theta)*cos(phi)*cos(psi))*((sin(phi)*sin(psi)*sin(theta) + cos(phi)*cos(psi))*cos(psi)*cos(theta) - (sin(phi)*sin(theta)*cos(psi) - sin(psi)*cos(phi))*sin(psi)*cos(theta)) - (-(sin(phi)*sin(psi) + sin(theta)*cos(phi)*cos(psi))*sin(psi)*cos(theta) + (-sin(phi)*cos(psi) + sin(psi)*sin(theta)*cos(phi))*cos(psi)*cos(theta))*(sin(phi)*sin(theta)*cos(psi) - sin(psi)*cos(phi)))*((sin(phi)*sin(theta)*cos(psi) - sin(psi)*cos(phi))*sin(theta) + sin(phi)*cos(psi)*cos(theta)^2)*cos(psi)*cos(theta))/((((sin(phi)*sin(psi) + sin(theta)*cos(phi)*cos(psi))*sin(theta) + cos(phi)*cos(psi)*cos(theta)^2)*((sin(phi)*sin(psi)*sin(theta) + cos(phi)*cos(psi))*cos(psi)*cos(theta) - (sin(phi)*sin(theta)*cos(psi) - sin(psi)*cos(phi))*sin(psi)*cos(theta)) - ((sin(phi)*sin(theta)*cos(psi) - sin(psi)*cos(phi))*sin(theta) + sin(phi)*cos(psi)*cos(theta)^2)*(-(sin(phi)*sin(psi) + sin(theta)*cos(phi)*cos(psi))*sin(psi)*cos(theta) + (-sin(phi)*cos(psi) + sin(psi)*sin(theta)*cos(phi))*cos(psi)*cos(theta)))*((sin(phi)*sin(psi)*sin(theta) + cos(phi)*cos(psi))*cos(psi)*cos(theta) - (sin(phi)*sin(theta)*cos(psi) - sin(psi)*cos(phi))*sin(psi)*cos(theta))*cos(psi)*cos(theta)), -((sin(phi)*sin(psi) + sin(theta)*cos(phi)*cos(psi))*((sin(phi)*sin(psi)*sin(theta) + cos(phi)*cos(psi))*cos(psi)*cos(theta) - (sin(phi)*sin(theta)*cos(psi) - sin(psi)*cos(phi))*sin(psi)*cos(theta)) - (-(sin(phi)*sin(psi) + sin(theta)*cos(phi)*cos(psi))*sin(psi)*cos(theta) + (-sin(phi)*cos(psi) + sin(psi)*sin(theta)*cos(phi))*cos(psi)*cos(theta))*(sin(phi)*sin(theta)*cos(psi) - sin(psi)*cos(phi)))/(((sin(phi)*sin(psi) + sin(theta)*cos(phi)*cos(psi))*sin(theta) + cos(phi)*cos(psi)*cos(theta)^2)*((sin(phi)*sin(psi)*sin(theta) + cos(phi)*cos(psi))*cos(psi)*cos(theta) - (sin(phi)*sin(theta)*cos(psi) - sin(psi)*cos(phi))*sin(psi)*cos(theta)) - ((sin(phi)*sin(theta)*cos(psi) - sin(psi)*cos(phi))*sin(theta) + sin(phi)*cos(psi)*cos(theta)^2)*(-(sin(phi)*sin(psi) + sin(theta)*cos(phi)*cos(psi))*sin(psi)*cos(theta) + (-sin(phi)*cos(psi) + sin(psi)*sin(theta)*cos(phi))*cos(psi)*cos(theta))), 0, 0, 0;(-(((sin(phi)*sin(psi) + sin(theta)*cos(phi)*cos(psi))*sin(theta) + cos(phi)*cos(psi)*cos(theta)^2)*((sin(phi)*sin(psi)*sin(theta) + cos(phi)*cos(psi))*cos(psi)*cos(theta) - (sin(phi)*sin(theta)*cos(psi) - sin(psi)*cos(phi))*sin(psi)*cos(theta)) - ((sin(phi)*sin(theta)*cos(psi) - sin(psi)*cos(phi))*sin(theta) + sin(phi)*cos(psi)*cos(theta)^2)*(-(sin(phi)*sin(psi) + sin(theta)*cos(phi)*cos(psi))*sin(psi)*cos(theta) + (-sin(phi)*cos(psi) + sin(psi)*sin(theta)*cos(phi))*cos(psi)*cos(theta)))*sin(psi)*cos(theta) - (((sin(phi)*sin(theta)*cos(psi) - sin(psi)*cos(phi))*sin(theta) + sin(phi)*cos(psi)*cos(theta)^2)*sin(psi)*cos(theta) + ((sin(phi)*sin(psi)*sin(theta) + cos(phi)*cos(psi))*cos(psi)*cos(theta) - (sin(phi)*sin(theta)*cos(psi) - sin(psi)*cos(phi))*sin(psi)*cos(theta))*sin(theta))*(-(sin(phi)*sin(psi) + sin(theta)*cos(phi)*cos(psi))*sin(psi)*cos(theta) + (-sin(phi)*cos(psi) + sin(psi)*sin(theta)*cos(phi))*cos(psi)*cos(theta)))/((((sin(phi)*sin(psi) + sin(theta)*cos(phi)*cos(psi))*sin(theta) + cos(phi)*cos(psi)*cos(theta)^2)*((sin(phi)*sin(psi)*sin(theta) + cos(phi)*cos(psi))*cos(psi)*cos(theta) - (sin(phi)*sin(theta)*cos(psi) - sin(psi)*cos(phi))*sin(psi)*cos(theta)) - ((sin(phi)*sin(theta)*cos(psi) - sin(psi)*cos(phi))*sin(theta) + sin(phi)*cos(psi)*cos(theta)^2)*(-(sin(phi)*sin(psi) + sin(theta)*cos(phi)*cos(psi))*sin(psi)*cos(theta) + (-sin(phi)*cos(psi) + sin(psi)*sin(theta)*cos(phi))*cos(psi)*cos(theta)))*((sin(phi)*sin(psi)*sin(theta) + cos(phi)*cos(psi))*cos(psi)*cos(theta) - (sin(phi)*sin(theta)*cos(psi) - sin(psi)*cos(phi))*sin(psi)*cos(theta))), ((((sin(phi)*sin(psi) + sin(theta)*cos(phi)*cos(psi))*sin(theta) + cos(phi)*cos(psi)*cos(theta)^2)*((sin(phi)*sin(psi)*sin(theta) + cos(phi)*cos(psi))*cos(psi)*cos(theta) - (sin(phi)*sin(theta)*cos(psi) - sin(psi)*cos(phi))*sin(psi)*cos(theta)) - ((sin(phi)*sin(theta)*cos(psi) - sin(psi)*cos(phi))*sin(theta) + sin(phi)*cos(psi)*cos(theta)^2)*(-(sin(phi)*sin(psi) + sin(theta)*cos(phi)*cos(psi))*sin(psi)*cos(theta) + (-sin(phi)*cos(psi) + sin(psi)*sin(theta)*cos(phi))*cos(psi)*cos(theta)))*cos(psi)*cos(theta) + ((sin(phi)*sin(theta)*cos(psi) - sin(psi)*cos(phi))*sin(theta) + sin(phi)*cos(psi)*cos(theta)^2)*(-(sin(phi)*sin(psi) + sin(theta)*cos(phi)*cos(psi))*sin(psi)*cos(theta) + (-sin(phi)*cos(psi) + sin(psi)*sin(theta)*cos(phi))*cos(psi)*cos(theta))*cos(psi)*cos(theta))/((((sin(phi)*sin(psi) + sin(theta)*cos(phi)*cos(psi))*sin(theta) + cos(phi)*cos(psi)*cos(theta)^2)*((sin(phi)*sin(psi)*sin(theta) + cos(phi)*cos(psi))*cos(psi)*cos(theta) - (sin(phi)*sin(theta)*cos(psi) - sin(psi)*cos(phi))*sin(psi)*cos(theta)) - ((sin(phi)*sin(theta)*cos(psi) - sin(psi)*cos(phi))*sin(theta) + sin(phi)*cos(psi)*cos(theta)^2)*(-(sin(phi)*sin(psi) + sin(theta)*cos(phi)*cos(psi))*sin(psi)*cos(theta) + (-sin(phi)*cos(psi) + sin(psi)*sin(theta)*cos(phi))*cos(psi)*cos(theta)))*((sin(phi)*sin(psi)*sin(theta) + cos(phi)*cos(psi))*cos(psi)*cos(theta) - (sin(phi)*sin(theta)*cos(psi) - sin(psi)*cos(phi))*sin(psi)*cos(theta))), -(-(sin(phi)*sin(psi) + sin(theta)*cos(phi)*cos(psi))*sin(psi)*cos(theta) + (-sin(phi)*cos(psi) + sin(psi)*sin(theta)*cos(phi))*cos(psi)*cos(theta))*cos(psi)*cos(theta)/(((sin(phi)*sin(psi) + sin(theta)*cos(phi)*cos(psi))*sin(theta) + cos(phi)*cos(psi)*cos(theta)^2)*((sin(phi)*sin(psi)*sin(theta) + cos(phi)*cos(psi))*cos(psi)*cos(theta) - (sin(phi)*sin(theta)*cos(psi) - sin(psi)*cos(phi))*sin(psi)*cos(theta)) - ((sin(phi)*sin(theta)*cos(psi) - sin(psi)*cos(phi))*sin(theta) + sin(phi)*cos(psi)*cos(theta)^2)*(-(sin(phi)*sin(psi) + sin(theta)*cos(phi)*cos(psi))*sin(psi)*cos(theta) + (-sin(phi)*cos(psi) + sin(psi)*sin(theta)*cos(phi))*cos(psi)*cos(theta))), 0, 0, 0;(((sin(phi)*sin(theta)*cos(psi) - sin(psi)*cos(phi))*sin(theta) + sin(phi)*cos(psi)*cos(theta)^2)*sin(psi)*cos(theta) + ((sin(phi)*sin(psi)*sin(theta) + cos(phi)*cos(psi))*cos(psi)*cos(theta) - (sin(phi)*sin(theta)*cos(psi) - sin(psi)*cos(phi))*sin(psi)*cos(theta))*sin(theta))/(((sin(phi)*sin(psi) + sin(theta)*cos(phi)*cos(psi))*sin(theta) + cos(phi)*cos(psi)*cos(theta)^2)*((sin(phi)*sin(psi)*sin(theta) + cos(phi)*cos(psi))*cos(psi)*cos(theta) - (sin(phi)*sin(theta)*cos(psi) - sin(psi)*cos(phi))*sin(psi)*cos(theta)) - ((sin(phi)*sin(theta)*cos(psi) - sin(psi)*cos(phi))*sin(theta) + sin(phi)*cos(psi)*cos(theta)^2)*(-(sin(phi)*sin(psi) + sin(theta)*cos(phi)*cos(psi))*sin(psi)*cos(theta) + (-sin(phi)*cos(psi) + sin(psi)*sin(theta)*cos(phi))*cos(psi)*cos(theta))), -((sin(phi)*sin(theta)*cos(psi) - sin(psi)*cos(phi))*sin(theta) + sin(phi)*cos(psi)*cos(theta)^2)*cos(psi)*cos(theta)/(((sin(phi)*sin(psi) + sin(theta)*cos(phi)*cos(psi))*sin(theta) + cos(phi)*cos(psi)*cos(theta)^2)*((sin(phi)*sin(psi)*sin(theta) + cos(phi)*cos(psi))*cos(psi)*cos(theta) - (sin(phi)*sin(theta)*cos(psi) - sin(psi)*cos(phi))*sin(psi)*cos(theta)) - ((sin(phi)*sin(theta)*cos(psi) - sin(psi)*cos(phi))*sin(theta) + sin(phi)*cos(psi)*cos(theta)^2)*(-(sin(phi)*sin(psi) + sin(theta)*cos(phi)*cos(psi))*sin(psi)*cos(theta) + (-sin(phi)*cos(psi) + sin(psi)*sin(theta)*cos(phi))*cos(psi)*cos(theta))), ((sin(phi)*sin(psi)*sin(theta) + cos(phi)*cos(psi))*cos(psi)*cos(theta) - (sin(phi)*sin(theta)*cos(psi) - sin(psi)*cos(phi))*sin(psi)*cos(theta))*cos(psi)*cos(theta)/(((sin(phi)*sin(psi) + sin(theta)*cos(phi)*cos(psi))*sin(theta) + cos(phi)*cos(psi)*cos(theta)^2)*((sin(phi)*sin(psi)*sin(theta) + cos(phi)*cos(psi))*cos(psi)*cos(theta) - (sin(phi)*sin(theta)*cos(psi) - sin(psi)*cos(phi))*sin(psi)*cos(theta)) - ((sin(phi)*sin(theta)*cos(psi) - sin(psi)*cos(phi))*sin(theta) + sin(phi)*cos(psi)*cos(theta)^2)*(-(sin(phi)*sin(psi) + sin(theta)*cos(phi)*cos(psi))*sin(psi)*cos(theta) + (-sin(phi)*cos(psi) + sin(psi)*sin(theta)*cos(phi))*cos(psi)*cos(theta))), 0, 0, 0;0, 0, 0, 1, (-(sin(phi)^2/cos(theta) + cos(phi)^2/cos(theta))*sin(phi)*sin(theta)/cos(theta) + (sin(phi)^2*sin(theta)/cos(theta) + sin(theta)*cos(phi)^2/cos(theta))*sin(phi)/cos(theta))/((sin(phi)^2/cos(theta) + cos(phi)^2/cos(theta))*cos(phi)), -(sin(phi)^2*sin(theta)/cos(theta) + sin(theta)*cos(phi)^2/cos(theta))/(sin(phi)^2/cos(theta) + cos(phi)^2/cos(theta));0, 0, 0, 0, cos(phi)/((sin(phi)^2/cos(theta) + cos(phi)^2/cos(theta))*cos(theta)), sin(phi)/(sin(phi)^2/cos(theta) + cos(phi)^2/cos(theta));0, 0, 0, 0, -sin(phi)/((sin(phi)^2/cos(theta) + cos(phi)^2/cos(theta))*cos(theta)), cos(phi)/(sin(phi)^2/cos(theta) + cos(phi)^2/cos(theta))]
